simulink model "c9_acc_via_delays1"  (R2022b)
settings: Solver=VariableStepAuto  StartTime=0  StopTime=30  MaxStep=1e-3  RelTol=1e-4
values from neighbouring files (symbols this model uses):
  L = Hbar'*W*Hbar    [c12_MultipleDelaysLMI.m]    (also in c14_bipartite_MWconsensus_animation.m = [A12+A13 -A12        -A13           Z                   Z   )
  tau = 1    [c12_delayAdaptive.m]
  x0 = 5    [c12_delayAdaptive.m]    (also in c14_bipartite_MWconsensus_animation.m = [x0;r/norm(r)]; c15_closed_model.m = 5*rand(15,1); c15_open_model.m = 5*rand(15,1))
settings Model: Creator=trinh  LastModifiedBy=trinh

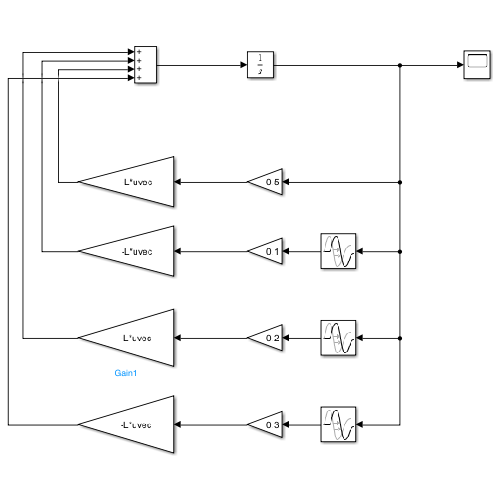
[thumbnail: Simulink's stored preview of the top-level diagram]
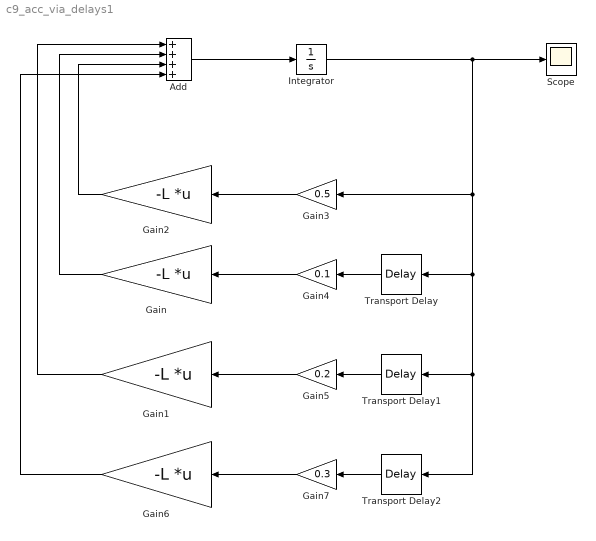
== system c9_acc_via_delays1 ==
  Add : Sum  Inputs=++++
  Gain{,1..2,6} (4 alike) : Gain  Gain=-L  Multiplication=Matrix(K*u) (u vector)
  Gain3 : Gain  Gain=0.5
  Gain4 : Gain  Gain=0.1
  Gain5 : Gain  Gain=0.2
  Gain7 : Gain  Gain=0.3
  Integrator : Integrator  InitialCondition=x0
  Scope : Scope
  Transport Delay : TransportDelay  DelayTime=tau  BufferSize=1024*8
  Transport Delay1 : TransportDelay  DelayTime=2*tau  BufferSize=1024*8
  Transport Delay2 : TransportDelay  DelayTime=2*tau  BufferSize=1024*8
  wires:
  Add/1 -> Integrator/1
  Transport Delay1/1 -> Gain5/1
  Gain/1 -> Add/2
  Gain1/1 -> Add/1
  Transport Delay/1 -> Gain4/1
  Gain2/1 -> Add/3
  Gain3/1 -> Gain2/1
  Gain4/1 -> Gain/1
  Gain5/1 -> Gain1/1
  Gain7/1 -> Gain6/1
  Integrator/1 -> Scope/1, Gain3/1, Transport Delay/1, Transport Delay2/1, Transport Delay1/1
  Transport Delay2/1 -> Gain7/1
  Gain6/1 -> Add/4
